simulink model "Simulation_ipmsm_velocity_control"  (R2023a)
settings: Solver=FixedStepDiscrete  StartTime=0.0  StopTime=2  FixedStep=Ts  RelTol=1e-3  EnableMultiTasking=on
PreLoadFcn:
  | ee_ipmsm_velocity_control_data;
StopFcn:
  | ee_addSimlogTimeStamp(bdroot)
undefined symbols (not defined in the file): Ld, Lq, p, psim, Ts, VDC_VECT, Vnom
libraries: nesl_utility x14, fl_lib x11, mcbcontrolslib x9, ee_lib x4, simulink x2, batteryecm_lib x1, eePmsmCurrentController x1, eeTransforms x1, eePmsmCurrentReferenceGen x1, eeVelocityController x1, eePwmGeneratorTwoLevel x1, SignalEditorBlockLib x1
(part 1 of 2)
CloseFcn:
  | try,close(h1_ee_ipmsm_velocity_control),end
  | clear h1_ee_ipmsm_velocity_control
  | 
  | clear simlog_ee_ipmsm_velocity_control
  | clear logsout_ee_ipmsm_velocity_control
  | 
  | clear Pmax Tmax p psim Ld Lq L0 Rs Jm
  | clear Cdc Vnom V1 AH0
  | clear Ts fsw Tsi Tso Kp_id Ki_id Kp_iq Ki_iq
  | clear numd_id dend_id numd_iq dend_iq
  | clear Kp_omega Ki_omega numd_omega dend_omega
  | clear ID_MAP IQ_MAP RPM_VECT TQ_VECT VDC_VECT
Description:
  | IPMSM Velocity Control
settings Model: Creator=The MathWorks, Inc.  LastModifiedBy=洲
settings SolverCC: AlgebraicLoopSolver=TrustRegion  MaxZcPerStep=1
settings DataIOCC: MaxDataPoints=210000  ReturnWorkspaceOutputs=off  SignalLoggingName=logsout_ee_ipmsm_velocity_control
settings OptimizationCC: ReuseModelBlockBuffer=off  LifeSpan=inf
settings DebuggingCC: MergeDetectMultiDrivingBlocksExec=none  UnconnectedInputMsg=warning  UnconnectedOutputMsg=warning  UnconnectedLineMsg=warning  SFUnexpectedBacktrackingDiag=warning  SFNoUnconditionalDefaultTransitionDiag=warning  SFExecutionAtInitializationDiag=none  ArithmeticOperatorsInVariantConditions=warning
settings ModelReferenceCC: EnableRefExpFcnMdlSchedulingChecks=on
settings SFSimCC: SimUseLocalCustomCode=off  CustomCodeUndefinedFunction=UseInterfaceOnly
settings RTWCC: RTWUseLocalCustomCode=off  DLArmComputeVersion=19.05
settings CodeAppCC: StateflowObjectComments=on
settings GRTTargetCC: TargetLangStandard=C89/C90 (ANSI)
settings ConfigComp: CovMetricSettings=dw  CovSaveCumulativeToWorkspaceVar=on  CovSaveSingleToWorkspaceVar=on  CovExternalEMLEnable=off
settings SimscapeCC: SimscapeNormalizeSystem=off  SimscapeLogType=all  SimscapeLogSimulationStatistics=on  SimscapeLogName=simlog_ee_ipmsm_velocity_control  SimscapeLogDataHistory=210000

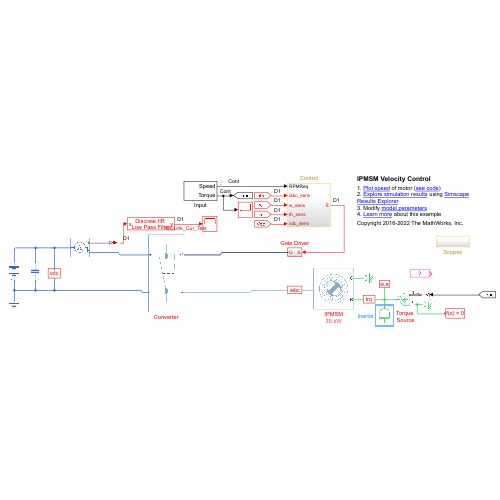
[thumbnail: Simulink's stored preview of the top-level diagram]
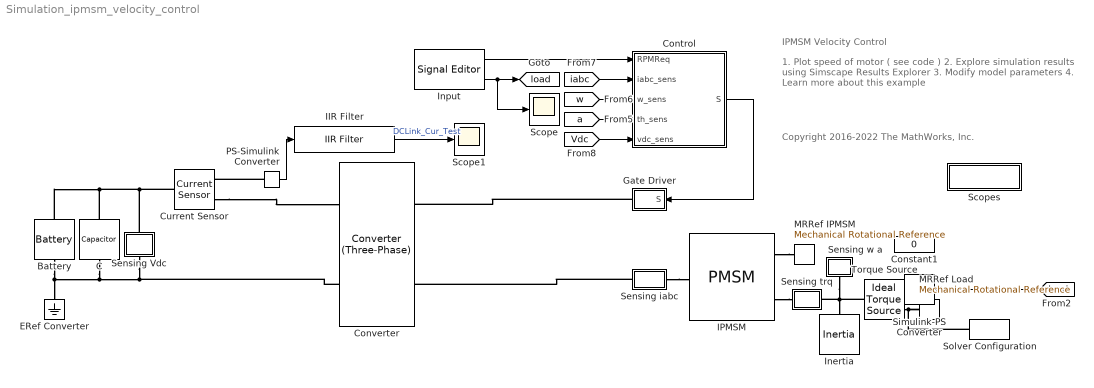
== system Simulation_ipmsm_velocity_control ==
  note: IPMSM Velocity Control
  note: 1. Plot speed of motor ( see code )
      | 2. Explore simulation results using Simscape Results Explorer
      | 3. Modify model parameters
      | 4. Learn more about this example
  note: Copyright 2016-2022 The MathWorks, Inc.
  Battery : batteryecm_lib/Battery  Vnom=Vnom V  prm_dir=1  R1_dis=2 Ohm  R1_ch=2 Ohm  R1=0.001 Ohm  prm_AH=1  AH=300 hr*A  V1=V1 V  AH1=100 hr*A  prm_R2=1  R2=2000 Ohm  Tmeas=298.15 K  charge_measurement_port=simscape.enum.battery.enable.no  prm_dyn=1  Rp1=0.005 Ohm  tau1=30 s  Rp2=0.005 Ohm  tau2=30 s  Rp3=0.005 Ohm  tau3=30 s  Rp4=0.005 Ohm  tau4=30 s  Rp5=0.005 Ohm  tau5=30 s  prm_fade=1  N_fade=100  AH_fade=45 hr*A  R1_fade=2.02 Ohm  R1_ch_fade=2.02 Ohm  V1_fade=10.35 V  prm_age=1  prm_age_OCV=1  OCV_age=0.9  SOC_age=60  Tmeas_age=298.15 K  delta_time_age_vec=[0] d  temperature_age_vec=[273] K  OCV_scaling_age=2.2134e6  OCV_offset_age=1.632e6  temp_exp_age=0.515833569 V  t_exp_age=0.75  Vnom_T2=12 V  R1_T2=2.2 Ohm  R1_T2_dis=2.2 Ohm  R1_T2_ch=2.2 Ohm  V1_T2=11.4 V  R2_T2=2200 Ohm  Rp1_T2=0.005 Ohm  tau1_T2=30 s  Rp2_T2=0.005 Ohm  tau2_T2=30 s  Rp3_T2=0.005 Ohm  tau3_T2=30 s  Rp4_T2=0.005 Ohm  tau4_T2=30 s  Rp5_T2=0.005 Ohm  tau5_T2=30 s  Tmeas2=273.15 K  thermal_port=simscape.enum.thermaleffects.omit  thermal_mass=30000 J/K  i_specify=off  i_priority=None  i=0 A  i_nominal_specify=off  i_nominal_unit=A  i_nominal_value=1  v_specify=off  v_priority=None  v=0 V  v_nominal_specify=off  v_nominal_unit=V  v_nominal_value=1  charge_specify=on  charge_priority=High  charge=AH0 hr*A  charge_nominal_specify=off  charge_nominal_unit=A*hr  charge_nominal_value=1  num_cycles_specify=off  num_cycles_priority=High  num_cycles=0  num_cycles_nominal_specify=off  num_cycles_nominal_unit=1  num_cycles_nominal_value=1  temperature_specify=off  temperature_priority=High  temperature=298.15 K  temperature_nominal_specify=off  temperature_nominal_unit=K  temperature_nominal_value=1
  C : fl_lib/Electrical/Electrical Elements/Capacitor  c=Cdc F  r=1e-6 Ohm  g=0 1/Ohm  i_specify=off  i_priority=None  i=0 A  i_nominal_specify=off  i_nominal_unit=A  i_nominal_value=1  v_specify=off  v_priority=None  v=0 V  v_nominal_specify=off  v_nominal_unit=V  v_nominal_value=1  vc_specify=on  vc_priority=None  vc=Vnom V  vc_nominal_specify=off  vc_nominal_unit=V  vc_nominal_value=1
  Constant1 : Constant  Value=0
  Control : Subsystem
  Converter : ee_lib/Semiconductors & Converters/Converters/Converter (Three-Phase)  port_option=ee.enum.threePhasePort.composite  device_type=3  K=0  Vf=0.8 V  Ron=0.001 Ohm  Rds=0.001 Ohm  Goff=1e-5 1/Ohm  Vgt=1 V  Vgt_off=-1 V  Ih=1 A  Vth=0.5 V  diode_param=2  diode_Vf=0.8 V  diode_Ron=0.001 Ohm  diode_Goff=1e-5 1/Ohm  diode_C=50 nF  diode_iRM=-235 A  diode_iF=300 A  diode_idot=-50 A/us  diode_trr_param=1  diode_trr_factor=3  diode_trr=15 us  diode_Qrr=1.5e+3 s*uA  snubber_type=0  Cs=1e-7 F  Rs=0.1 Ohm
  Current Sensor : fl_lib/Electrical/Electrical Sensors/Current Sensor
  ERef Converter : fl_lib/Electrical/Electrical Elements/Electrical Reference
  Gate Driver : Subsystem
  IIR Filter : mcbcontrolslib/IIR Filter  VariantControl=Low Pass Filter  VariantSelect=Low-pass  Filter_constant=0.001  advancedSettings=off  Ts=50e-6  cutOff_freq=3.1863
      settings: LibrarySourceBlock=mcbhdllib/Signal Management/IIR Filter
  IPMSM : ee_lib/Electromechanical/Permanent Magnet/PMSM  port_option=ee.enum.threePhasePort.composite  winding_type=ee.enum.statorconnection.wye  machine_param=ee.enum.pmsm.parameterization.constant  nPolePairs=p  pmflux_param=1  pm_flux_linkage=psim Wb  torque_constant=0.18 N*m/A  back_emf_constant=0.18 V/(rad/s)  stator_param=1  Ld=Ld H  Lq=Lq H  idVec=[-200, 0, 200] A  iqVec=[-200, 0, 200] A  LdMatrix=0.0002 * ones(3, 3) H  LqMatrix=0.0002 * ones(3, 3) H  PmMatrix=0.1 * ones(3, 3) Wb  ktMatrix=0.18 * ones(3, 3) N*m/A  keMatrix=0.18 * ones(3, 3) V/(rad/s)  L0=L0 H  Ls=0.0002 H  Lm=0.00002 H  Ms=0.00002 H  Rs=Rs Ohm  zero_sequence=ee.enum.park.zerosequence.exclude  axes_param=ee.enum.rotorangle.daxis  loss_param=ee.enum.ironloss.none  losses_oc=[0, 0, 0] W  losses_sc=[0, 0, 0] W  f_losses=60 Hz  Isc_losses=95 A  J=0 kg*m^2  lam=0 N*m/(rad/s)  i_d_specify=off  i_d_priority=None  i_d=0 A  i_d_nominal_specify=off  i_d_nominal_unit=A  i_d_nominal_value=1  i_q_specify=off  i_q_priority=None  i_q=0 A  i_q_nominal_specify=off  i_q_nominal_unit=A  i_q_nominal_value=1  torque_specify=off  torque_priority=None  torque=0 N*m  torque_nominal_specify=off  torque_nominal_unit=N*m  torque_nominal_value=1  angular_velocity_specify=on  angular_velocity_priority=None  angular_velocity=0 rpm  angular_velocity_nominal_specify=off  angular_velocity_nominal_unit=rpm  angular_velocity_nominal_value=1  angular_position_specify=on  angular_position_priority=High  angular_position=0 rad  angular_position_nominal_specify=off  angular_position_nominal_unit=deg  angular_position_nominal_value=1  alpha=3.93e-3 1/K  alpha_flux=-0.001 1/K  Tmeas=298.15 K  stator_thermal_mass=100 J/K  rotor_thermal_mass=200 J/K  Rm_percent_rotor=90  Rd_percent_rotor=30  temperatureA_specify=off  temperatureA_priority=High  temperatureA=25 degC  temperatureA_nominal_specify=off  temperatureA_nominal_unit=degC  temperatureA_nominal_value=1  temperatureB_specify=off  temperatureB_priority=High  temperatureB=25 degC  temperatureB_nominal_specify=off  temperatureB_nominal_unit=degC  temperatureB_nominal_value=1  temperatureC_specify=off  temperatureC_priority=High  temperatureC=25 degC  temperatureC_nominal_specify=off  temperatureC_nominal_unit=degC  temperatureC_nominal_value=1  temperatureR_specify=off  temperatureR_priority=High  temperatureR=25 degC  temperatureR_nominal_specify=off  temperatureR_nominal_unit=degC  temperatureR_nominal_value=1
      settings: AttributesFormatString=35 kW  InternalSimscapePortConfiguration="{\"Bottom\":[],\"Left\":[{\"id\":\"N\",\"label\":\"~\",\"type\":\"foundation.electrical.three_phase\"}],\"Right\":[{\"id\":\"R\",\"label\":\"R\",\"type\":\"foundation.mechanical.rotational.rotational\"},{\"id\":\"C\",\"label\":\"C\",\"type\":\"foundation.mechanical.rotational.rotational\"}],\"Top\":[]}"
  Inertia : fl_lib/Mechanical/Rotational Elements/Inertia  inertia=Jm kg*m^2  num_ports=foundation.enum.numPorts2.one  w_specify=on  w_priority=High  w=0 rpm  w_nominal_specify=off  w_nominal_unit=rad/s  w_nominal_value=1  t_specify=off  t_priority=High  t=0 N*m  t_nominal_specify=off  t_nominal_unit=N*m  t_nominal_value=1
  Input : SignalEditorBlockLib/Signal Editor  FileName=ee_ipmsm_velocity_control_Input.mat  ActiveScenario=Test_1  ActiveSignal=Torque  IsBus=off  OutputBusObjectStr=Bus: BusObject  SampleTime=0  OutputAfterFinalValue=Extrapolation  Unit=inherit  PreserveSignalName=on  ApplySigPropsToAllScenarios=on
  MRRef IPMSM : fl_lib/Mechanical/Rotational Elements/Mechanical Rotational Reference
  MRRef Load : fl_lib/Mechanical/Rotational Elements/Mechanical Rotational Reference
  PS-Simulink Converter : nesl_utility/PS-Simulink Converter  PhysicalDomain=network_engine_domain  SubClassName=ps_output  LeftPortType=input  RightPortType=output  PseudoPeriodic=off  Frequencies=[]  VectorFormat=inherit  Unit=inherit  AffineConversion=off
  Scope : Scope
  Scope1 : Scope
  Scopes : Subsystem
  Sensing Vdc : Subsystem
      mask Display: disp('vdc')
  Sensing trq : Subsystem
      mask Display: disp('trq')
  Sensing w a : Subsystem
      mask Display: disp('w,a')
  Sensing iabc : Subsystem
      mask Display: disp('iabc')
  Simulink-PS Converter : nesl_utility/Simulink-PS Converter  PhysicalDomain=network_engine_domain  SubClassName=ps_input  LeftPortType=input  RightPortType=output  PseudoPeriodic=off  Frequencies=[]  NoiseDistribution=none  NoiseParameters=[]  Unit=N*m  AffineConversion=off  FilteringAndDerivatives=zero  SimscapeFilterOrder=1  InputFilterTimeConstant=0.001  UdotUserProvided=1
  Solver Configuration : nesl_utility/Solver Configuration  PhysicalDomain=network_engine_domain  SubClassName=solver  LeftPortType=input  RightPortType=generic  Tones=[]  Harmonics=[]  SimulateNoise=off  Profile=off  UseLocalSampling=off  EnableSwitchedLinearOptims=on  FrequencyDomain=off  UseCCode=off  RelTol=0.001  AbsTol=1e-06  MinStep=1e-09  ToWorkspace=off  RevertToSquareIcSolve=off  NumHomotopyIterations=100  PhasorMode=off  PhasorModeNumHarmonics=1  ConsistencySolver=NEWTON_FTOL  IndexReductionMethod=DerivativeReplacement  DoDC=off  ResidualTolerance=1e-9  ConsistencyTolSource=GLOBAL  ConsistencyAbsTol=0.001  ConsistencyRelTol=0.001  ConsistencyTolFactor=0.001  UseLocalSolver=on  LocalSolverChoice=NE_BACKWARD_EULER_ADVANCER  ResolveIndetEquations=on  FunctionEvalNumThread=1  LocalSolverSampleTime=Ts  DoFixedCost=on  MaxNonlinIter=5  MaxModeIter=2  ComputeImpulses=off  ImpulseIterations=2  LinearAlgebra=auto  LinearAlgebraNumThread=0  EquationFormulation=NE_TIME_EF  DelaysMemoryBudget=1024  AutomaticFiltering=on  FilteringTimeConstant=0.001  PartitionStorageMethod=AS_NEEDED  PartitionMemoryBudget=1024  PartitionMethod=FAST
  Torque Source : fl_lib/Mechanical/Mechanical Sources/Ideal Torque Source
  tag scope: load=global
  wires:
  Control/1(S) -> Gate Driver/1(S)
  [Vdc] -> Control/5(vdc_sens)
  [iabc] -> Control/2(iabc_sens)
  [w] -> Control/3(w_sens)
  [a] -> Control/4(th_sens)
  Input/2 -> [load], Scope/1
  Input/1 -> Control/1(RPMReq)
  PS-Simulink Converter/1 -> IIR Filter/1
  IIR Filter/1 -> Scope1/1  "DCLink_Cur_Test"
  [load] -> Simulink-PS Converter/1
  connections:
  Sensing Vdc/LConn1 -- Current Sensor/LConn1 -- C/LConn1 -- Battery/LConn1
  Torque Source/LConn1 -- Sensing trq/RConn1 -- Inertia/LConn1 -- Sensing w a/LConn1
  Gate Driver/RConn1 -- Converter/LConn1
  Torque Source/RConn1 -- Simulink-PS Converter/RConn1
  Torque Source/RConn2 -- Solver Configuration/RConn1 -- MRRef Load/LConn1
  Sensing iabc/LConn1 -- Converter/LConn2
  Sensing iabc/RConn1 -- IPMSM/LConn1
  IPMSM/RConn2 -- MRRef IPMSM/LConn1
  IPMSM/RConn1 -- Sensing trq/LConn1
  Battery/RConn1 -- C/RConn1 -- Sensing Vdc/RConn1 -- Converter/RConn2 -- ERef Converter/LConn1
  Current Sensor/RConn2 -- Converter/RConn1
  PS-Simulink Converter/LConn1 -- Current Sensor/RConn1

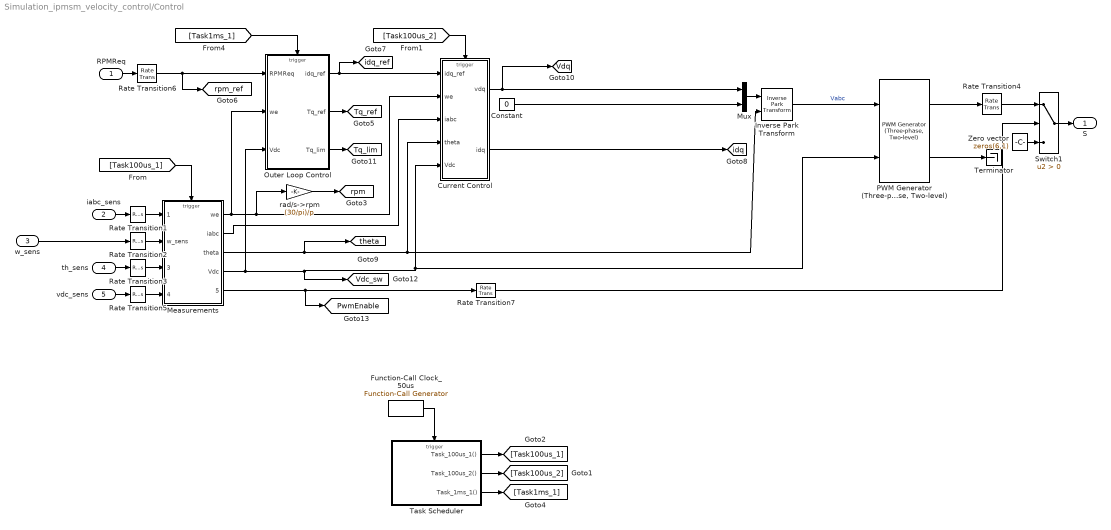
== system Simulation_ipmsm_velocity_control/Control ==
  RPMReq : Inport
  iabc_sens : Inport  Port=2
  w_sens : Inport  Port=3
  th_sens : Inport  Port=4
  vdc_sens : Inport  Port=5
  Constant : Constant  Value=0  SampleTime=-1
  Current Control : Subsystem
  Function-Call Clock_50us : simulink/Ports & Subsystems/Function-Call Generator  sample_time=5e-5  numberOfIterations=1  DisallowWideOutput=off
  Inverse Park Transform : eeTransforms/Inverse Park Transform  AxisAlignment=D-axis  PowerInvariant=off
  Measurements : Subsystem
  Mux : Mux  Inputs=2
  Outer Loop Control : Subsystem
  "PWM Generator (Three-phase, Two-level)" : eePwmGeneratorTwoLevel/PWM Generator (Three-phase, Two-level)  PWMMode=Continuous PWM (CPWM)  CPWMMode=SVM: space vector modulation  DPWMMode=60 DPWM: 60 degree discontinuous PWM  fsw=fsw  Ts=Ts
  Rate Transition{1..7} (7 alike) : RateTransition
  Switch1 : Switch  Criteria=u2 > Threshold  SaturateOnIntegerOverflow=off  InputSameDT=off
  Task Scheduler : Stateflow chart  TreatAsAtomicUnit=on
  Terminator : Terminator
  Zero vector : Constant  Value=zeros(6,1)
  rad/s->rpm : Gain  Gain=(30/pi)/p
  S : Outport  VectorParamsAs1DForOutWhenUnconnected=off
  tag scope: PwmEnable=global, Tq_lim=global, Tq_ref=global, Vdc_sw=global, Vdq=global, idq=global, idq_ref=global, rpm=global, rpm_ref=global, theta=global
  wires:
  [Task100us_1] -> Measurements/Trigger
  [Task100us_2] -> Current Control/Trigger
  Current Control/1(vdq) -> [Vdq], Mux/1
  Measurements/2(iabc) -> Current Control/3(iabc)
  Measurements/3(theta) -> [theta], Inverse Park Transform/2, Current Control/4(theta)
  "PWM Generator (Three-phase, Two-level)"/1 -> Rate Transition4/1
  Inverse Park Transform/1 -> "PWM Generator (Three-phase, Two-level)"/1  "Vabc"
  iabc_sens/1 -> Rate Transition1/1
  w_sens/1 -> Rate Transition2/1
  th_sens/1 -> Rate Transition3/1
  vdc_sens/1 -> Rate Transition5/1
  Outer Loop Control/1(idq_ref) -> [idq_ref], Current Control/1(idq_ref)
  RPMReq/1 -> Rate Transition6/1
  "PWM Generator (Three-phase, Two-level)"/2 -> Terminator/1
  Rate Transition1/1 -> Measurements/1(iabc_sens)
  Rate Transition2/1 -> Measurements/2(w_sens)
  Rate Transition3/1 -> Measurements/3(th_sens)
  Rate Transition5/1 -> Measurements/4(Vdc_sens)
  Rate Transition6/1 -> [rpm_ref], Outer Loop Control/1(RPMReq)
  Measurements/4(Vdc) -> [Vdc_sw], "PWM Generator (Three-phase, Two-level)"/2, Current Control/5(Vdc), Outer Loop Control/3(Vdc)
  Function-Call Clock_50us/1 -> Task Scheduler/Trigger
  Task Scheduler/3(Task_1ms_1()) -> [Task1ms_1]
  Task Scheduler/2(Task_100us_2()) -> [Task100us_2]
  Task Scheduler/1(Task_100us_1()) -> [Task100us_1]
  Outer Loop Control/2(Tq_ref) -> [Tq_ref]
  Measurements/1(we) -> Current Control/2(we), rad/s->rpm/1, Outer Loop Control/2(we)
  rad/s->rpm/1 -> [rpm]
  Current Control/2(idq) -> [idq]
  Outer Loop Control/3(Tq_lim) -> [Tq_lim]
  Switch1/1 -> S/1
  Rate Transition4/1 -> Switch1/1
  Measurements/5(PwmEnable) -> [PwmEnable], Rate Transition7/1
  Zero vector/1 -> Switch1/3
  Rate Transition7/1 -> Switch1/2
  [Task1ms_1] -> Outer Loop Control/Trigger
  Mux/1 -> Inverse Park Transform/1
  Constant/1 -> Mux/2

== system Simulation_ipmsm_velocity_control/Gate Driver ==
  S : Inport
  Demux : Demux  Outputs=6
  Simulink-PS Converter{1..6} (6 alike) : nesl_utility/Simulink-PS Converter  PhysicalDomain=network_engine_domain  SubClassName=ps_input  LeftPortType=input  RightPortType=output  PseudoPeriodic=off  Frequencies=[]  NoiseDistribution=none  NoiseParameters=[]  Unit=1  AffineConversion=off  FilteringAndDerivatives=zero  SimscapeFilterOrder=1  InputFilterTimeConstant=0.001  UdotUserProvided=1
  Six-Pulse Gate Multiplexer : ee_lib/Semiconductors & Converters/Converters/Six-Pulse Gate Multiplexer  port_option=ee.enum.controlport.ps
  G : PMIOPort  Side=Right
  wires:
  Demux/1 -> Simulink-PS Converter1/1
  S/1 -> Demux/1
  Demux/4 -> Simulink-PS Converter4/1
  Demux/2 -> Simulink-PS Converter2/1
  Demux/3 -> Simulink-PS Converter3/1
  Demux/5 -> Simulink-PS Converter5/1
  Demux/6 -> Simulink-PS Converter6/1
  connections:
  Six-Pulse Gate Multiplexer/RConn1 -- G/RConn1
  Simulink-PS Converter1/RConn1 -- Six-Pulse Gate Multiplexer/LConn1
  Simulink-PS Converter3/RConn1 -- Six-Pulse Gate Multiplexer/LConn3
  Simulink-PS Converter5/RConn1 -- Six-Pulse Gate Multiplexer/LConn5
  Simulink-PS Converter6/RConn1 -- Six-Pulse Gate Multiplexer/LConn6
  Simulink-PS Converter4/RConn1 -- Six-Pulse Gate Multiplexer/LConn4
  Simulink-PS Converter2/RConn1 -- Six-Pulse Gate Multiplexer/LConn2

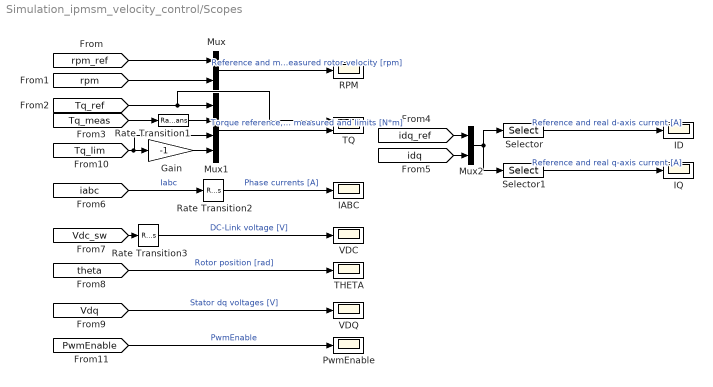
== system Simulation_ipmsm_velocity_control/Scopes ==
  Gain : Gain  Gain=-1
  IABC : Scope
  ID : Scope
  IQ : Scope
  Mux : Mux  Inputs=2
  Mux1 : Mux
  Mux2 : Mux  Inputs=2
  PwmEnable : Scope
  RPM : Scope
  Rate Transition1 : RateTransition
  Rate Transition2 : RateTransition  OutPortSampleTime=1e-4
  Rate Transition3 : RateTransition  OutPortSampleTime=1e-4
  Selector : Selector  InputPortWidth=4  IndexOptions=Index vector (dialog)  Indices=[1 3]  OutputSizes=1
  Selector1 : Selector  InputPortWidth=4  IndexOptions=Index vector (dialog)  Indices=[2 4]  OutputSizes=1
  THETA : Scope
  TQ : Scope  NumInputPorts=2
  VDC : Scope
  VDQ : Scope
  wires:
  [rpm] -> Mux/2
  Selector1/1 -> IQ/1  "Reference and real q-axis current [A]"
  Mux2/1 -> Selector1/1, Selector/1
  Gain/1 -> Mux1/4
  Rate Transition3/1 -> VDC/1  "DC-Link voltage [V]"
  [Vdc_sw] -> Rate Transition3/1
  [idq_ref] -> Mux2/1
  [PwmEnable] -> PwmEnable/1  "PwmEnable"
  [Tq_ref] -> TQ/1, Mux1/1
  Rate Transition2/1 -> IABC/1  "Phase currents [A]"
  [idq] -> Mux2/2
  [rpm_ref] -> Mux/1
  [iabc] -> Rate Transition2/1  "Iabc"
  [Tq_meas] -> Rate Transition1/1
  [Vdq] -> VDQ/1  "Stator dq voltages [V]"
  Selector/1 -> ID/1  "Reference and real d-axis current [A]"
  [Tq_lim] -> Mux1/3, Gain/1
  Mux1/1 -> TQ/2  "Torque reference, measured and limits [N*m]"
  [theta] -> THETA/1  "Rotor position [rad]"
  Rate Transition1/1 -> Mux1/2
  Mux/1 -> RPM/1  "Reference and measured rotor velocity [rpm]"

== system Simulation_ipmsm_velocity_control/Sensing Vdc ==
  PS-Simulink Converter4 : nesl_utility/PS-Simulink Converter  PhysicalDomain=network_engine_domain  SubClassName=ps_output  LeftPortType=input  RightPortType=output  PseudoPeriodic=off  Frequencies=[]  VectorFormat=1-D array  Unit=V  AffineConversion=off
  Voltage Sensor : fl_lib/Electrical/Electrical Sensors/Voltage Sensor
  + : PMIOPort  Side=Left
  - : PMIOPort  Port=2  Side=Right
  tag scope: Vdc=global
  wires:
  PS-Simulink Converter4/1 -> [Vdc]
  connections:
  Voltage Sensor/LConn1 -- +/RConn1
  Voltage Sensor/RConn2 -- -/RConn1
  PS-Simulink Converter4/LConn1 -- Voltage Sensor/RConn1

== system Simulation_ipmsm_velocity_control/Sensing trq ==
  PS-Simulink Converter3 : nesl_utility/PS-Simulink Converter  PhysicalDomain=network_engine_domain  SubClassName=ps_output  LeftPortType=input  RightPortType=output  PseudoPeriodic=off  Frequencies=[]  VectorFormat=1-D array  Unit=N*m  AffineConversion=off
  Torque Sensor : fl_lib/Mechanical/Mechanical Sensors/Ideal Torque Sensor
  R : PMIOPort  Side=Left
  C : PMIOPort  Port=2  Side=Right
  tag scope: Tq_meas=global
  wires:
  PS-Simulink Converter3/1 -> [Tq_meas]
  connections:
  Torque Sensor/RConn1 -- C/RConn1
  Torque Sensor/RConn2 -- PS-Simulink Converter3/LConn1
  Torque Sensor/LConn1 -- R/RConn1

== system Simulation_ipmsm_velocity_control/Sensing w a ==
  MRRef : fl_lib/Mechanical/Rotational Elements/Mechanical Rotational Reference
  Motion Sensor : fl_lib/Mechanical/Mechanical Sensors/Ideal Rotational Motion Sensor  reference=foundation.enum.MeasurementReference.difference  acceleration_port=false  velocity_port=true  position_port=true  wrap_angle=simscape.enum.onoff.off  offset=0 deg
  PS-Simulink Converter1 : nesl_utility/PS-Simulink Converter  PhysicalDomain=network_engine_domain  SubClassName=ps_output  LeftPortType=input  RightPortType=output  PseudoPeriodic=off  Frequencies=[]  VectorFormat=1-D array  Unit=rad/s  AffineConversion=off
  PS-Simulink Converter2 : nesl_utility/PS-Simulink Converter  PhysicalDomain=network_engine_domain  SubClassName=ps_output  LeftPortType=input  RightPortType=output  PseudoPeriodic=off  Frequencies=[]  VectorFormat=1-D array  Unit=rad  AffineConversion=off
  Scope : Scope
  R : PMIOPort  Side=Left
  tag scope: a=global, w=global
  wires:
  PS-Simulink Converter1/1 -> [w]  "eSpd"
  PS-Simulink Converter2/1 -> [a]
  connections:
  R/RConn1 -- Motion Sensor/LConn1
  Motion Sensor/RConn2 -- PS-Simulink Converter1/LConn1
  MRRef/LConn1 -- Motion Sensor/RConn1
  Motion Sensor/RConn3 -- PS-Simulink Converter2/LConn1

== system Simulation_ipmsm_velocity_control/Sensing iabc ==
  Current Sensor : ee_lib/Sensors & Transducers/Current Sensor (Three-Phase)
  PS-Simulink Converter : nesl_utility/PS-Simulink Converter  PhysicalDomain=network_engine_domain  SubClassName=ps_output  LeftPortType=input  RightPortType=output  PseudoPeriodic=off  Frequencies=[]  VectorFormat=1-D array  Unit=A  AffineConversion=off
  1 : PMIOPort  Side=Left
  2 : PMIOPort  Port=2  Side=Right
  tag scope: iabc=global
  wires:
  PS-Simulink Converter/1 -> [iabc]
  connections:
  1/RConn1 -- Current Sensor/LConn1
  2/RConn1 -- Current Sensor/RConn2
  Current Sensor/RConn1 -- PS-Simulink Converter/LConn1

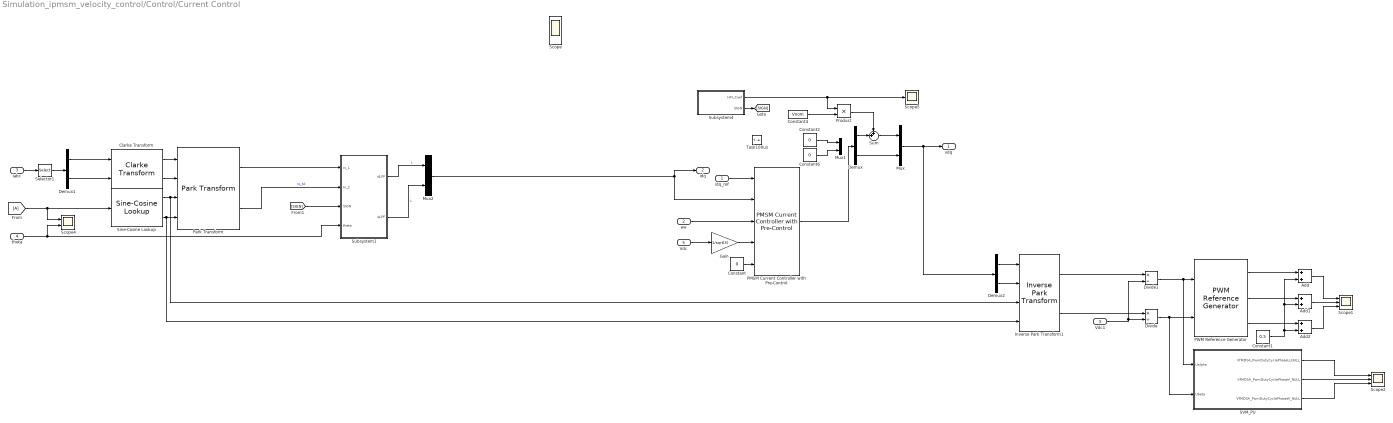
== system Simulation_ipmsm_velocity_control/Control/Current Control ==
  idq_ref : Inport
  we : Inport  Port=2
  iabc : Inport  Port=3
  theta : Inport  Port=4
  Vdc : Inport  Port=5
  Task100us : TriggerPort  TriggerType=function-call  VariantControl=Variant  PortDimensions=1
  Add : Sum
  Add1 : Sum
  Add2 : Sum
  Clarke Transform : mcbcontrolslib/Clarke Transform  VariantControl=Variant2
      settings: LibrarySourceBlock=mcblib/Controls/Math Transforms/Clarke Transform
  Constant : Constant  Value=0  SampleTime=-1
  Constant1 : Constant  Value=0.5
  Constant2 : Constant  Value=0
  Constant4 : Constant  Value=Vnom
  Constant6 : Constant  Value=0
  Demux : Demux  Outputs=2
  Demux1 : Demux  Outputs=2
  Demux2 : Demux  Outputs=2
  Divide : Product  Inputs=*/
  Divide1 : Product  Inputs=*/
  From : From
  Gain : Gain  Gain=1/sqrt(3)
  Inverse Park Transform1 : mcbcontrolslib/Inverse Park Transform  AxisAlignment=D-axis
      settings: LibrarySourceBlock=mcblib/Controls/Math Transforms/Inverse Park Transform
  Mux : Mux  Inputs=2
  Mux1 : Mux  Inputs=2
  Mux2 : Mux  Inputs=2
  PMSM Current Controller with Pre-Control : eePmsmCurrentController/PMSM Current Controller with Pre-Control  Kp_id=Kp_id  Ki_id=Ki_id  Kaw_id=1  Kp_iq=Kp_iq  Ki_iq=Ki_iq  Kaw_iq=1  Ts=-1  Tsd=Tsi  AxisPrio=D-axis  ActZC=on  ActFF=on  idVect=[-200, 0, 200]  iqVect=[-200, 0, 200]  LdMatrix=Ld * ones(3, 3)  LqMatrix=Lq * ones(3, 3)  psimMatrix=psim * ones(3, 3)
  PWM Reference Generator : mcbcontrolslib/PWM Reference Generator  inSignal=Valphabeta  modType=SVM: space vector modulation
      settings: LibrarySourceBlock=mcblib/Controls/Math Transforms/PWM Reference Generator
  Park Transform : mcbcontrolslib/Park Transform  AxisAlignment=D-axis
      settings: LibrarySourceBlock=mcblib/Controls/Math Transforms/Park Transform
  Product : Product
  SVM_PU : Subsystem  TreatAsAtomicUnit=on  RTWFcnName=SVPWM_Calc
      settings: RTWSystemCode=Nonreusable function  RTWFcnNameOpts=User specified
  Scope : Scope  NumInputPorts=4
  Scope1 : Scope  NumInputPorts=3
  Scope2 : Scope  NumInputPorts=3
  Scope4 : Scope  NumInputPorts=2
  Scope5 : Scope
  Selector1 : Selector  InputPortWidth=3  IndexOptions=Index vector (dialog)  Indices=[1 2]  OutputSizes=1
  Sine-Cosine Lookup : mcbcontrolslib/Sine-Cosine Lookup  AngleInput=Radians  N_points=4095
      settings: LibrarySourceBlock=mcblib/Controls/Math Transforms/Sine-Cosine Lookup
  Subsystem1 : Subsystem
  Subsystem4 : Subsystem
  Sum : Sum  Inputs=++|
  Vdc1 : InportShadow  Port=5
  vdq : Outport  VectorParamsAs1DForOutWhenUnconnected=off
  idq : Outport  Port=2  VectorParamsAs1DForOutWhenUnconnected=off
  wires:
  Vdc/1 -> Gain/1
  we/1 -> PMSM Current Controller with Pre-Control/3
  idq_ref/1 -> PMSM Current Controller with Pre-Control/1
  Constant/1 -> PMSM Current Controller with Pre-Control/5
  Mux2/1 -> idq/1, PMSM Current Controller with Pre-Control/2
  Gain/1 -> PMSM Current Controller with Pre-Control/4
  iabc/1 -> Selector1/1
  Selector1/1 -> Demux1/1
  Demux1/1 -> Clarke Transform/1
  Demux1/2 -> Clarke Transform/2
  Clarke Transform/1 -> Park Transform/1
  Clarke Transform/2 -> Park Transform/2
  Sine-Cosine Lookup/1 -> Inverse Park Transform1/3, Park Transform/3
  Sine-Cosine Lookup/2 -> Inverse Park Transform1/4, Park Transform/4
  Mux/1 -> vdq/1, Demux2/1
  Park Transform/1 -> Subsystem1/1(In_1)
  Park Transform/2 -> Subsystem1/2(In_2)  "Iq_bk"
  From/1 -> Scope4/1, Sine-Cosine Lookup/1
  Demux2/1 -> Inverse Park Transform1/1
  Demux2/2 -> Inverse Park Transform1/2
  Vdc1/1 -> Divide1/2, Divide/2
  Inverse Park Transform1/1 -> Divide1/1
  Divide1/1 -> SVM_PU/1(Ualpha), PWM Reference Generator/1
  Divide/1 -> PWM Reference Generator/2, SVM_PU/2(Ubeta)
  Inverse Park Transform1/2 -> Divide/1
  PWM Reference Generator/1 -> Add/1
  PWM Reference Generator/2 -> Add1/1
  PWM Reference Generator/3 -> Add2/1
  Constant1/1 -> Add/2, Add1/2, Add2/2
  Add/1 -> Scope1/1
  Add1/1 -> Scope1/2
  Add2/1 -> Scope1/3
  SVM_PU/2(VfMDSA_PwmDutyCyclePhaseV_NULL) -> Scope2/2
  SVM_PU/1(VfMDSA_PwmDutyCyclePhaseU_NULL) -> Scope2/1
  SVM_PU/3(VfMDSA_PwmDutyCyclePhaseW_NULL) -> Scope2/3
  Product/1 -> Sum/1
  Constant4/1 -> Product/2
  Subsystem4/1(HFI_Coef) -> Scope5/1, Product/1
  theta/1 -> Subsystem1/4(theta), Scope4/2
  Sum/1 -> Mux/1
  Demux/1 -> Sum/2
  Demux/2 -> Mux/2
  Constant2/1 -> Mux1/1
  Constant6/1 -> Mux1/2
  PMSM Current Controller with Pre-Control/1 -> Demux/1
  Subsystem1/1(dLPF) -> Mux2/1  "L"
  Subsystem1/2(qLPF) -> Mux2/2  "L"
  Subsystem4/2(SIGN) -> [SIGN]
  [SIGN] -> Subsystem1/3(SIGN)

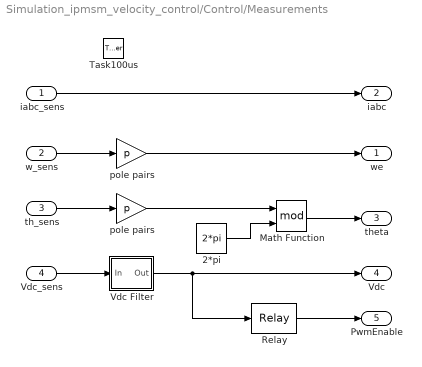
== system Simulation_ipmsm_velocity_control/Control/Measurements ==
  iabc_sens : Inport
  w_sens : Inport  Port=2
  th_sens : Inport  Port=3
  Vdc_sens : Inport  Port=4
  Task100us : TriggerPort  TriggerType=function-call  VariantControl=Variant  PortDimensions=1
  2*pi : Constant  Value=2*pi  SampleTime=-1
  Math Function : Math  Operator=mod  SignedPower=on
  Relay : Relay  OnSwitchValue=VDC_VECT(1)  OffSwitchValue=0.5*VDC_VECT(1)
  Vdc Filter : Subsystem  mask(Discrete first-order filter (Low-pass)){T=0.005, Ts=1e-4}
      mask prompts: T "Time constant (s):"; Ts "Sample time (s):"
      mask help: This block implements a discrete low-pass filter. To calculate the coefficients, the block discretises a continuous low-pass filter using the Tustin method.
      mask init:
      | num = [ Ts/(2*T + Ts), Ts/(2*T + Ts)];
      | den = [ 1, -(2*T - Ts)/(2*T + Ts)];
  pole pairs : Gain  Gain=p
  "pole pairs " : Gain  Gain=p
  we : Outport  VectorParamsAs1DForOutWhenUnconnected=off
  iabc : Outport  Port=2  VectorParamsAs1DForOutWhenUnconnected=off
  theta : Outport  Port=3  VectorParamsAs1DForOutWhenUnconnected=off
  Vdc : Outport  Port=4  VectorParamsAs1DForOutWhenUnconnected=off
  PwmEnable : Outport  Port=5  VectorParamsAs1DForOutWhenUnconnected=off
  wires:
  pole pairs/1 -> we/1
  Vdc_sens/1 -> Vdc Filter/1(In)
  th_sens/1 -> "pole pairs "/1
  w_sens/1 -> pole pairs/1
  iabc_sens/1 -> iabc/1
  "pole pairs "/1 -> Math Function/1
  2*pi/1 -> Math Function/2
  Math Function/1 -> theta/1
  Relay/1 -> PwmEnable/1
  Vdc Filter/1(Out) -> Relay/1, Vdc/1

== system Simulation_ipmsm_velocity_control/Control/Outer Loop Control ==
  RPMReq : Inport
  we : Inport  Port=2
  Vdc : Inport  Port=3
  Task1ms : TriggerPort  TriggerType=function-call  VariantControl=Variant  PortDimensions=1
  Constant : Constant  Value=0  SampleTime=-1
  PMSM Current Reference Generator : eePmsmCurrentReferenceGen/PMSM Current Reference Generator  Vnom=Vnom  Pmax=Pmax  Tmax=Tmax  Ts=-1  RefType=Lookup-table based  rpmVec=RPM_VECT  TqVec=TQ_VECT  VdcVec=VDC_VECT  PWMMode=SVM: space vector modulation  ModFactor=1  idMatrix=ID_MAP  iqMatrix=IQ_MAP  p=8  psim=0.04  Ld=0.00024  Lq=0.00029  Rs=0.01  RefExpEnable=0
  Velocity Controller : eeVelocityController/Velocity Controller  CtrlType=P-PI control  Kp_w=Kp_omega  Ki_w=Ki_omega  Kv_w=Kp_omega  Kaw_w=100  Ts=-1  Tsd=Tso  ActZC=on
  elec->mech : Gain  Gain=1/p
  rpm->rad/s : Gain  Gain=(pi/30)
  idq_ref : Outport  VectorParamsAs1DForOutWhenUnconnected=off
  Tq_ref : Outport  Port=2  VectorParamsAs1DForOutWhenUnconnected=off
  Tq_lim : Outport  Port=3  VectorParamsAs1DForOutWhenUnconnected=off
  wires:
  rpm->rad/s/1 -> Velocity Controller/1
  Velocity Controller/1 -> PMSM Current Reference Generator/1
  RPMReq/1 -> rpm->rad/s/1
  we/1 -> elec->mech/1
  Vdc/1 -> PMSM Current Reference Generator/3
  PMSM Current Reference Generator/1 -> idq_ref/1
  PMSM Current Reference Generator/2 -> Tq_ref/1, Velocity Controller/3
  PMSM Current Reference Generator/3 -> Tq_lim/1
  elec->mech/1 -> PMSM Current Reference Generator/2, Velocity Controller/2
  Constant/1 -> Velocity Controller/4

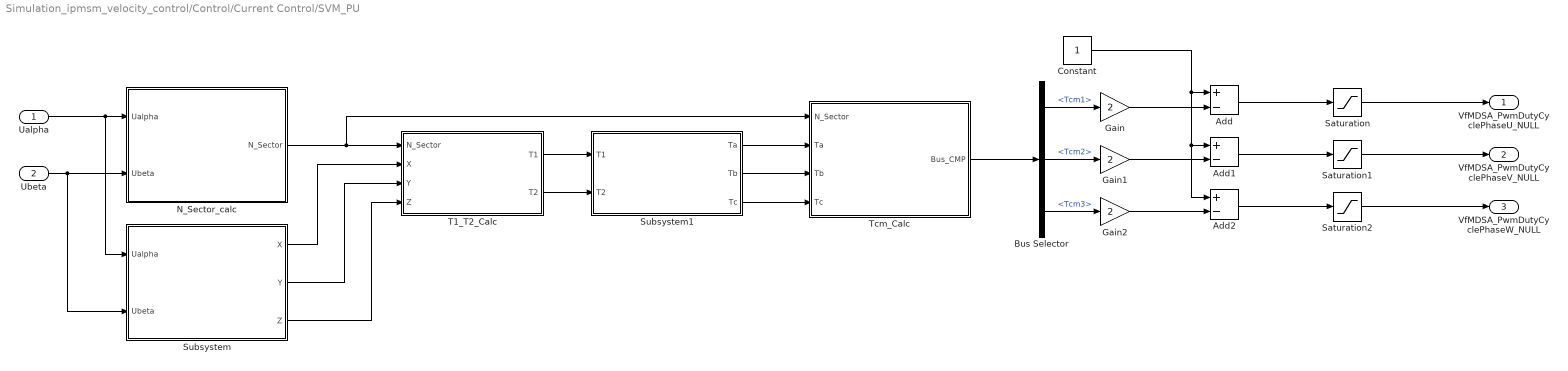
== system Simulation_ipmsm_velocity_control/Control/Current Control/SVM_PU ==
  Ualpha : Inport
  Ubeta : Inport  Port=2
  Add : Sum  Inputs=+-
  Add1 : Sum  Inputs=+-
  Add2 : Sum  Inputs=+-
  Bus Selector : BusSelector  OutputSignals=Tcm1,Tcm2,Tcm3
  Constant : Constant  OutDataTypeStr=single
  Gain : Gain  Gain=2
  Gain1 : Gain  Gain=2
  Gain2 : Gain  Gain=2
  N_Sector_calc : Subsystem
  Saturation : Saturate  UpperLimit=1  LowerLimit=0
  Saturation1 : Saturate  UpperLimit=1  LowerLimit=0
  Saturation2 : Saturate  UpperLimit=1  LowerLimit=0
  Subsystem : Subsystem
  Subsystem1 : Subsystem
  T1_T2_Calc : Subsystem
  Tcm_Calc : Subsystem
  VfMDSA_PwmDutyCyclePhaseU_NULL : Outport  OutMin=0  OutMax=1
  VfMDSA_PwmDutyCyclePhaseV_NULL : Outport  Port=2  OutMin=0  OutMax=1
  VfMDSA_PwmDutyCyclePhaseW_NULL : Outport  Port=3  OutMin=0  OutMax=1
  wires:
  Ualpha/1 -> Subsystem/1(Ualpha), N_Sector_calc/1(Ualpha)
  Ubeta/1 -> Subsystem/2(Ubeta), N_Sector_calc/2(Ubeta)
  N_Sector_calc/1(N_Sector) -> Tcm_Calc/1(N_Sector), T1_T2_Calc/1(N_Sector)
  Subsystem/1(X) -> T1_T2_Calc/2(X)
  Subsystem/2(Y) -> T1_T2_Calc/3(Y)
  Subsystem/3(Z) -> T1_T2_Calc/4(Z)
  Subsystem1/1(Ta) -> Tcm_Calc/2(Ta)
  Subsystem1/2(Tb) -> Tcm_Calc/3(Tb)
  Subsystem1/3(Tc) -> Tcm_Calc/4(Tc)
  Tcm_Calc/1(Bus_CMP) -> Bus Selector/1
  T1_T2_Calc/1(T1) -> Subsystem1/1(T1)
  T1_T2_Calc/2(T2) -> Subsystem1/2(T2)
  Bus Selector/1 -> Gain/1  "<Tcm1>"
  Bus Selector/2 -> Gain1/1  "<Tcm2>"
  Bus Selector/3 -> Gain2/1  "<Tcm3>"
  Constant/1 -> Add2/1, Add1/1, Add/1
  Gain/1 -> Add/2
  Gain1/1 -> Add1/2
  Gain2/1 -> Add2/2
  Add/1 -> Saturation/1
  Add1/1 -> Saturation1/1
  Add2/1 -> Saturation2/1
  Saturation/1 -> VfMDSA_PwmDutyCyclePhaseU_NULL/1
  Saturation1/1 -> VfMDSA_PwmDutyCyclePhaseV_NULL/1
  Saturation2/1 -> VfMDSA_PwmDutyCyclePhaseW_NULL/1

== system Simulation_ipmsm_velocity_control/Control/Current Control/Subsystem1 ==
  In_1 : Inport
  In_2 : Inport  Port=2
  SIGN : Inport  Port=3
  theta : Inport  Port=4
  Inverse Park Transform : mcbcontrolslib/Inverse Park Transform  AxisAlignment=D-axis
      settings: LibrarySourceBlock=mcblib/Controls/Math Transforms/Inverse Park Transform
  Scope : Scope  NumInputPorts=3
  Sine-Cosine Lookup : mcbcontrolslib/Sine-Cosine Lookup  AngleInput=Radians  N_points=4095
      settings: LibrarySourceBlock=mcblib/Controls/Math Transforms/Sine-Cosine Lookup
  Subsystem : Subsystem
  Subsystem2 : Subsystem
  Subsystem3 : Subsystem
  atan2 : mcbcontrolslib/atan2  outputUnit=Radians
      settings: LibrarySourceBlock=mcblib/Controls/Math Transforms/atan2
  dLPF : Outport
  qLPF : Outport  Port=2
  wires:
  Subsystem2/1(LPF) -> dLPF/1
  Subsystem3/2(LPF) -> qLPF/1
  In_1/1 -> Subsystem2/1(In_1)
  In_2/1 -> Subsystem3/1(In_2)
  Subsystem2/2(HPF) -> Subsystem/1(dHPF)
  Subsystem3/1(HPF) -> Subsystem/2(qHPF)
  SIGN/1 -> Subsystem/3(SIGN)
  Subsystem/1(delta_Id) -> Inverse Park Transform/1
  Subsystem/2(delta_Iq) -> Inverse Park Transform/2
  Sine-Cosine Lookup/2 -> Inverse Park Transform/4
  Sine-Cosine Lookup/1 -> Inverse Park Transform/3
  theta/1 -> Sine-Cosine Lookup/1
  Inverse Park Transform/1 -> Scope/1, atan2/1
  Inverse Park Transform/2 -> atan2/2, Scope/2
  atan2/1 -> Scope/3

== system Simulation_ipmsm_velocity_control/Control/Current Control/Subsystem4 ==
  Subsystem : Subsystem
  HFI_Coef : Outport
  SIGN : Outport  Port=2
  wires:
  Subsystem/1(HFI_Coef) -> HFI_Coef/1
  Subsystem/2(SIGN) -> SIGN/1

== system Simulation_ipmsm_velocity_control/Control/Measurements/Vdc Filter ==
  In : Inport
  Discrete Transfer Fcn : DiscreteTransferFcn  Numerator=num  Denominator=den
  Out : Outport  VectorParamsAs1DForOutWhenUnconnected=off
  wires:
  Discrete Transfer Fcn/1 -> Out/1
  In/1 -> Discrete Transfer Fcn/1

== system Simulation_ipmsm_velocity_control/Control/Current Control/SVM_PU/N_Sector_calc ==
  Ualpha : Inport
  Ubeta : Inport  Port=2
  N_calc : Subsystem
  Uref_Calc : Subsystem
  N_Sector : Outport
  wires:
  Uref_Calc/2(Uref2) -> N_calc/2(Uref2)
  Ualpha/1 -> Uref_Calc/1(Ualpha)
  Ubeta/1 -> Uref_Calc/2(Ubeta)
  Uref_Calc/3(Uref3) -> N_calc/3(Uref3)
  N_calc/1(N_Sector) -> N_Sector/1
  Uref_Calc/1(Uref1) -> N_calc/1(Uref1)

== system Simulation_ipmsm_velocity_control/Control/Current Control/SVM_PU/Subsystem ==
  Ualpha : Inport
  Ubeta : Inport  Port=2
  Add1 : Sum
  Add2 : Sum  Inputs=-+
  ConstanT1 : Constant  Value=2  OutDataTypeStr=single
  ConstanT2 : Constant  Value=sqrt(3)/2  OutDataTypeStr=single
  Constant : Constant  Value=3/2  OutDataTypeStr=single
  ProducT1 : Product
  ProducT2 : Product
  Product : Product
  X : Outport
  Y : Outport  Port=2
  Z : Outport  Port=3
  wires:
  Ualpha/1 -> Product/1
  Constant/1 -> Product/2
  ProducT1/1 -> X/1
  ConstanT1/1 -> ProducT1/2
  Ubeta/1 -> ProducT2/1
  Add1/1 -> Y/1
  Product/1 -> Add2/1, Add1/1
  ProducT2/1 -> ProducT1/1, Add2/2, Add1/2
  ConstanT2/1 -> ProducT2/2
  Add2/1 -> Z/1

== system Simulation_ipmsm_velocity_control/Control/Current Control/SVM_PU/Subsystem1 ==
  T1 : Inport
  T2 : Inport  Port=2
  Add : Sum  Inputs=+--
  Add1 : Sum  Inputs=++-
  Add2 : Sum  Inputs=+++
  Constant : Constant  Value=1/4  OutDataTypeStr=single
  Gain1 : Gain  Gain=1/4
  Gain2 : Gain  Gain=1/4
  Ta : Outport
  Tb : Outport  Port=2
  Tc : Outport  Port=3
  wires:
  T1/1 -> Gain1/1
  T2/1 -> Gain2/1
  Constant/1 -> Add2/1, Add1/1, Add/1
  Add/1 -> Ta/1
  Gain1/1 -> Add2/2, Add1/2, Add/2
  Gain2/1 -> Add1/3, Add2/3, Add/3
  Add1/1 -> Tb/1
  Add2/1 -> Tc/1

== system Simulation_ipmsm_velocity_control/Control/Current Control/SVM_PU/T1_T2_Calc ==
  N_Sector : Inport
  X : Inport  Port=2
  Y : Inport  Port=3
  Z : Inport  Port=4
  Subsystem1 : Subsystem
  Subsystem2 : Subsystem
  T4_T6 : Subsystem  Commented=on
  T1 : Outport
  T2 : Outport  Port=2
  wires:
  X/1 -> Subsystem1/2(X)
  Z/1 -> Subsystem1/4(Z)
  N_Sector/1 -> Subsystem1/1(N_Sector)
  Y/1 -> Subsystem1/3(Y)
  Subsystem1/1(Bus_T4T6) -> Subsystem2/1(Bus_T4T6)
  Subsystem2/1(T1) -> T1/1
  Subsystem2/2(T2) -> T2/1

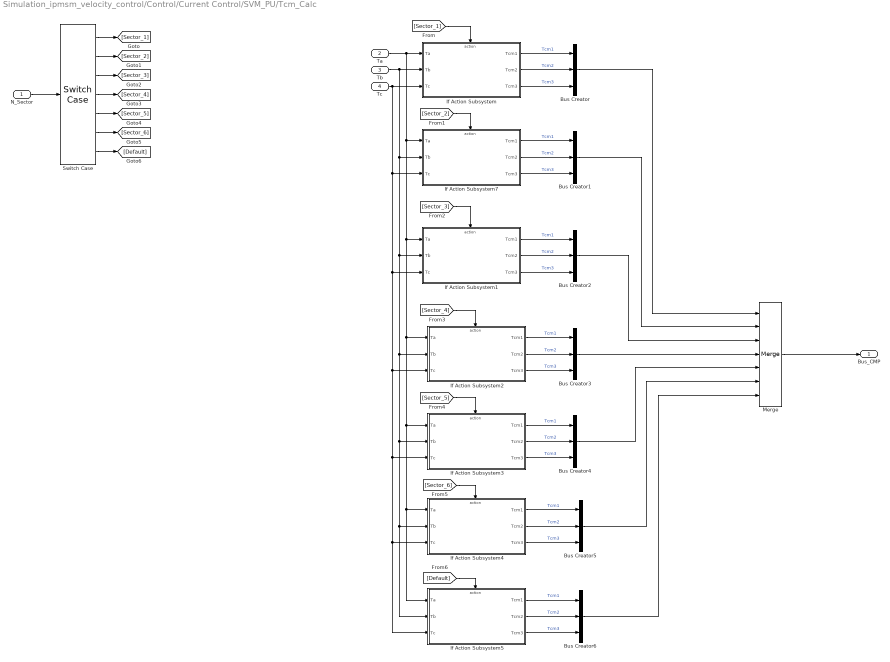
== system Simulation_ipmsm_velocity_control/Control/Current Control/SVM_PU/Tcm_Calc ==
  N_Sector : Inport
  Ta : Inport  Port=2
  Tb : Inport  Port=3
  Tc : Inport  Port=4
  Bus Creator{,1..6} (7 alike) : BusCreator  Inputs=3
  If Action Subsystem : Subsystem  TreatAsAtomicUnit=on
  If Action Subsystem1 : Subsystem  TreatAsAtomicUnit=on
  If Action Subsystem2 : Subsystem  TreatAsAtomicUnit=on
  If Action Subsystem3 : Subsystem  TreatAsAtomicUnit=on
  If Action Subsystem4 : Subsystem  TreatAsAtomicUnit=on
  If Action Subsystem5 : Subsystem  TreatAsAtomicUnit=on
  If Action Subsystem7 : Subsystem  TreatAsAtomicUnit=on
  Merge : Merge  Inputs=7
  Switch Case : SwitchCase  CaseConditions={1,2,3,4,5,6}
  Bus_CMP : Outport
  wires:
  Switch Case/1 -> [Sector_1]
  Switch Case/2 -> [Sector_2]
  Switch Case/4 -> [Sector_4]
  Switch Case/6 -> [Sector_6]
  Switch Case/3 -> [Sector_3]
  N_Sector/1 -> Switch Case/1
  Switch Case/7 -> [Default]
  Switch Case/5 -> [Sector_5]
  [Sector_1] -> If Action Subsystem/Action
  [Sector_2] -> If Action Subsystem7/Action
  [Sector_4] -> If Action Subsystem2/Action
  [Sector_3] -> If Action Subsystem1/Action
  [Sector_6] -> If Action Subsystem4/Action
  [Sector_5] -> If Action Subsystem3/Action
  [Default] -> If Action Subsystem5/Action
  Tb/1 -> If Action Subsystem5/2(Tb), If Action Subsystem4/2(Tb), If Action Subsystem3/2(Tb), If Action Subsystem2/2(Tb), If Action Subsystem1/2(Tb), If Action Subsystem7/2(Tb), If Action Subsystem/2(Tb)
  Tc/1 -> If Action Subsystem/3(Tc), If Action Subsystem5/3(Tc), If Action Subsystem4/3(Tc), If Action Subsystem3/3(Tc), If Action Subsystem2/3(Tc), If Action Subsystem1/3(Tc), If Action Subsystem7/3(Tc)
  Ta/1 -> If Action Subsystem5/1(Ta), If Action Subsystem4/1(Ta), If Action Subsystem3/1(Ta), If Action Subsystem2/1(Ta), If Action Subsystem1/1(Ta), If Action Subsystem7/1(Ta), If Action Subsystem/1(Ta)
  Merge/1 -> Bus_CMP/1
  If Action Subsystem/1(Tcm1) -> Bus Creator/1  "Tcm1"
  If Action Subsystem/2(Tcm2) -> Bus Creator/2  "Tcm2"
  If Action Subsystem/3(Tcm3) -> Bus Creator/3  "Tcm3"
  If Action Subsystem7/1(Tcm1) -> Bus Creator1/1  "Tcm1"
  If Action Subsystem7/3(Tcm3) -> Bus Creator1/3  "Tcm3"
  If Action Subsystem7/2(Tcm2) -> Bus Creator1/2  "Tcm2"
  If Action Subsystem1/1(Tcm1) -> Bus Creator2/1  "Tcm1"
  If Action Subsystem1/3(Tcm3) -> Bus Creator2/3  "Tcm3"
  If Action Subsystem1/2(Tcm2) -> Bus Creator2/2  "Tcm2"
  If Action Subsystem2/1(Tcm1) -> Bus Creator3/1  "Tcm1"
  If Action Subsystem2/3(Tcm3) -> Bus Creator3/3  "Tcm3"
  If Action Subsystem2/2(Tcm2) -> Bus Creator3/2  "Tcm2"
  If Action Subsystem3/1(Tcm1) -> Bus Creator4/1  "Tcm1"
  If Action Subsystem3/3(Tcm3) -> Bus Creator4/3  "Tcm3"
  If Action Subsystem3/2(Tcm2) -> Bus Creator4/2  "Tcm2"
  If Action Subsystem4/1(Tcm1) -> Bus Creator5/1  "Tcm1"
  If Action Subsystem4/3(Tcm3) -> Bus Creator5/3  "Tcm3"
  If Action Subsystem4/2(Tcm2) -> Bus Creator5/2  "Tcm2"
  If Action Subsystem5/1(Tcm1) -> Bus Creator6/1  "Tcm1"
  If Action Subsystem5/3(Tcm3) -> Bus Creator6/3  "Tcm3"
  If Action Subsystem5/2(Tcm2) -> Bus Creator6/2  "Tcm2"
  Bus Creator/1 -> Merge/1
  Bus Creator1/1 -> Merge/2
  Bus Creator2/1 -> Merge/3
  Bus Creator3/1 -> Merge/4
  Bus Creator4/1 -> Merge/5
  Bus Creator5/1 -> Merge/6
  Bus Creator6/1 -> Merge/7

== system Simulation_ipmsm_velocity_control/Control/Current Control/Subsystem1/Subsystem ==
  dHPF : Inport
  qHPF : Inport  Port=2
  SIGN : Inport  Port=3
  Add : Sum  Inputs=+-
  Add1 : Sum  Inputs=+-
  Delay : Delay  DelayLength=1
  Delay1 : Delay  DelayLength=1
  Product : Product
  Product1 : Product
  delta_Id : Outport
  delta_Iq : Outport  Port=2
  wires:
  dHPF/1 -> Delay/1, Add/1
  Delay/1 -> Add/2
  Add/1 -> Product/1
  qHPF/1 -> Delay1/1, Add1/1
  Delay1/1 -> Add1/2
  Add1/1 -> Product1/2
  SIGN/1 -> Product1/1, Product/2
  Product/1 -> delta_Id/1
  Product1/1 -> delta_Iq/1

== system Simulation_ipmsm_velocity_control/Control/Current Control/Subsystem1/Subsystem2 ==
  In_1 : Inport
  Add3 : Sum  Inputs=+-
  Constant7 : Constant  Value=0.0001
  Constant8 : Constant  Value=20
  HPF_Calc : Subsystem
  LPF : Outport
  HPF : Outport  Port=2
  wires:
  In_1/1 -> Add3/1, HPF_Calc/1(In1)
  Constant8/1 -> HPF_Calc/2(VfHpf_FilterCornerFreq_Hz)
  HPF_Calc/1(HPF) -> Add3/2, HPF/1
  Constant7/1 -> HPF_Calc/3(VfHpf_FilterTs_s)
  Add3/1 -> LPF/1

== system Simulation_ipmsm_velocity_control/Control/Current Control/Subsystem1/Subsystem3 ==
  In_2 : Inport
  Add3 : Sum  Inputs=+-
  Constant7 : Constant  Value=0.0001
  Constant8 : Constant  Value=20
  HPF_Calc : Subsystem
  HPF : Outport
  LPF : Outport  Port=2
  wires:
  In_2/1 -> Add3/1, HPF_Calc/1(In1)
  Constant8/1 -> HPF_Calc/2(VfHpf_FilterCornerFreq_Hz)
  HPF_Calc/1(HPF) -> Add3/2, HPF/1
  Constant7/1 -> HPF_Calc/3(VfHpf_FilterTs_s)
  Add3/1 -> LPF/1

== system Simulation_ipmsm_velocity_control/Control/Current Control/Subsystem4/Subsystem ==
  Compare To Constant : simulink/Logic and Bit Operations/Compare To Constant  relop=>  const=0  OutDataTypeStr=boolean
  Constant : Constant  OutDataTypeStr=single
  Constant1 : Constant  Value=-1  OutDataTypeStr=single
  Constant2 : Constant  Value=0.02
  Delay1 : Delay  DelayLength=1  InitialCondition=1
  Gain : Gain  Gain=-1
  Product1 : Product
  Switch : Switch  Criteria=u2 > Threshold  SaturateOnIntegerOverflow=off  InputSameDT=off
  HFI_Coef : Outport
  SIGN : Outport  Port=2
  wires:
  Constant/1 -> Switch/1
  Constant1/1 -> Switch/3
  Delay1/1 -> Gain/1, Compare To Constant/1  "HFI_Last_Coef"
  Gain/1 -> Product1/1, Delay1/1
  Compare To Constant/1 -> Switch/2
  Constant2/1 -> Product1/2
  Product1/1 -> HFI_Coef/1
  Switch/1 -> SIGN/1

== system Simulation_ipmsm_velocity_control/Control/Current Control/SVM_PU/N_Sector_calc/N_calc ==
  Uref1 : Inport
  Uref2 : Inport  Port=2
  Uref3 : Inport  Port=3
  Add : Sum  Inputs=+++
  ConstanT1 : Constant  Value=0  OutDataTypeStr=single
  Constant : Constant  OutDataTypeStr=single
  Gain : Gain
  Gain1 : Gain  Gain=2
  Gain2 : Gain  Gain=4
  Switch : Switch  Criteria=u2 > Threshold  SaturateOnIntegerOverflow=off  InputSameDT=off
  Switch1 : Switch  Criteria=u2 > Threshold  SaturateOnIntegerOverflow=off  InputSameDT=off
  Switch2 : Switch  Criteria=u2 > Threshold  SaturateOnIntegerOverflow=off  InputSameDT=off
  N_Sector : Outport
  wires:
  Uref1/1 -> Switch/2
  Uref2/1 -> Switch1/2
  Uref3/1 -> Switch2/2
  ConstanT1/1 -> Switch2/3, Switch/3, Switch1/3
  Constant/1 -> Switch2/1, Switch1/1, Switch/1
  Switch1/1 -> Gain1/1
  Switch/1 -> Gain/1
  Switch2/1 -> Gain2/1
  Add/1 -> N_Sector/1
  Gain/1 -> Add/1
  Gain1/1 -> Add/2
  Gain2/1 -> Add/3

== system Simulation_ipmsm_velocity_control/Control/Current Control/SVM_PU/N_Sector_calc/Uref_Calc ==
  Ualpha : Inport
  Ubeta : Inport  Port=2
  Add : Sum  Inputs=+-
  Add1 : Sum  Inputs=--
  ConstanT1 : Constant  Value=sqrt(1)/2  OutDataTypeStr=single
  Constant : Constant  Value=sqrt(3)/2  OutDataTypeStr=single
  ProducT1 : Product
  Product : Product
  Signal Copy : SignalConversion  OverrideOpt=off
  Uref1 : Outport
  Uref2 : Outport  Port=2
  Uref3 : Outport  Port=3
  wires:
  Ubeta/1 -> ProducT1/1, Signal Copy/1
  Signal Copy/1 -> Uref1/1
  Ualpha/1 -> Product/1
  Constant/1 -> Product/2
  ConstanT1/1 -> ProducT1/2
  Product/1 -> Add1/1, Add/1
  ProducT1/1 -> Add1/2, Add/2
  Add/1 -> Uref2/1
  Add1/1 -> Uref3/1

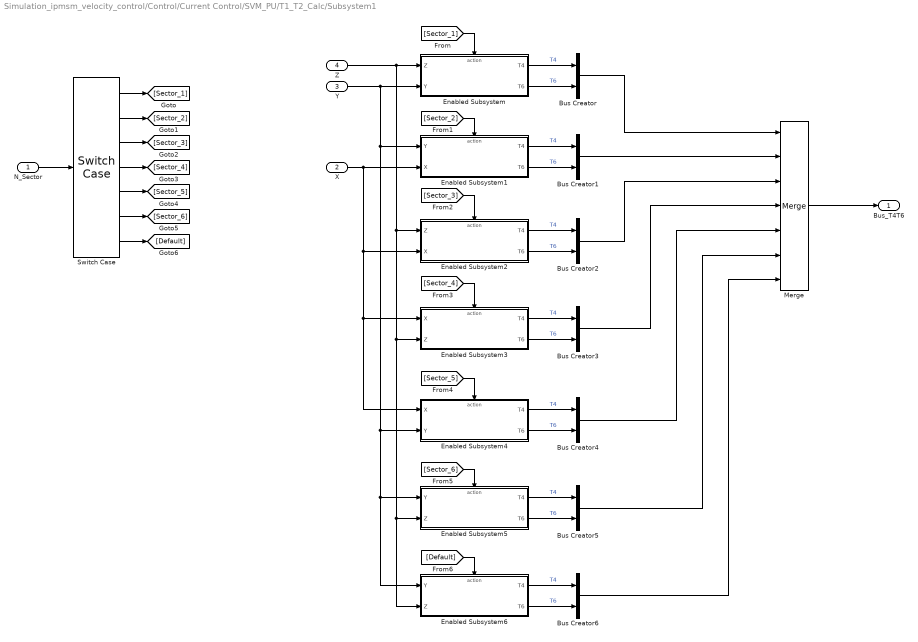
== system Simulation_ipmsm_velocity_control/Control/Current Control/SVM_PU/T1_T2_Calc/Subsystem1 ==
  N_Sector : Inport
  X : Inport  Port=2
  Y : Inport  Port=3
  Z : Inport  Port=4
  Bus Creator{,1..6} (7 alike) : BusCreator  Inputs=2
  Enabled Subsystem : Subsystem  TreatAsAtomicUnit=on
  Enabled Subsystem1 : Subsystem  TreatAsAtomicUnit=on
  Enabled Subsystem2 : Subsystem  TreatAsAtomicUnit=on
  Enabled Subsystem3 : Subsystem  TreatAsAtomicUnit=on
  Enabled Subsystem4 : Subsystem  TreatAsAtomicUnit=on
  Enabled Subsystem5 : Subsystem  TreatAsAtomicUnit=on
  Enabled Subsystem6 : Subsystem  TreatAsAtomicUnit=on
  Merge : Merge  Inputs=7
  Switch Case : SwitchCase  CaseConditions={1,2,3,4,5,6}
  Bus_T4T6 : Outport
  wires:
  N_Sector/1 -> Switch Case/1
  Switch Case/1 -> [Sector_1]
  Switch Case/2 -> [Sector_2]
  Switch Case/3 -> [Sector_3]
  Switch Case/4 -> [Sector_4]
  Switch Case/5 -> [Sector_5]
  Switch Case/6 -> [Sector_6]
  Switch Case/7 -> [Default]
  [Sector_1] -> Enabled Subsystem/Action
  Y/1 -> Enabled Subsystem6/1(Y), Enabled Subsystem5/1(Y), Enabled Subsystem4/2(Y), Enabled Subsystem1/1(Y), Enabled Subsystem/2(Y)
  Z/1 -> Enabled Subsystem3/2(Z), Enabled Subsystem6/2(Z), Enabled Subsystem5/2(Z), Enabled Subsystem2/1(Z), Enabled Subsystem/1(Z)
  [Sector_2] -> Enabled Subsystem1/Action
  X/1 -> Enabled Subsystem4/1(X), Enabled Subsystem3/1(X), Enabled Subsystem2/2(X), Enabled Subsystem1/2(X)
  [Sector_3] -> Enabled Subsystem2/Action
  [Sector_4] -> Enabled Subsystem3/Action
  [Sector_5] -> Enabled Subsystem4/Action
  [Sector_6] -> Enabled Subsystem5/Action
  [Default] -> Enabled Subsystem6/Action
  Enabled Subsystem/1(T4) -> Bus Creator/1  "T4"
  Enabled Subsystem/2(T6) -> Bus Creator/2  "T6"
  Enabled Subsystem1/2(T6) -> Bus Creator1/2  "T6"
  Enabled Subsystem1/1(T4) -> Bus Creator1/1  "T4"
  Enabled Subsystem2/1(T4) -> Bus Creator2/1  "T4"
  Enabled Subsystem3/1(T4) -> Bus Creator3/1  "T4"
  Enabled Subsystem2/2(T6) -> Bus Creator2/2  "T6"
  Enabled Subsystem3/2(T6) -> Bus Creator3/2  "T6"
  Enabled Subsystem4/1(T4) -> Bus Creator4/1  "T4"
  Enabled Subsystem5/1(T4) -> Bus Creator5/1  "T4"
  Enabled Subsystem4/2(T6) -> Bus Creator4/2  "T6"
  Enabled Subsystem5/2(T6) -> Bus Creator5/2  "T6"
  Enabled Subsystem6/1(T4) -> Bus Creator6/1  "T4"
  Enabled Subsystem6/2(T6) -> Bus Creator6/2  "T6"
  Bus Creator/1 -> Merge/1
  Bus Creator1/1 -> Merge/2
  Bus Creator2/1 -> Merge/3
  Bus Creator3/1 -> Merge/4
  Bus Creator4/1 -> Merge/5
  Bus Creator5/1 -> Merge/6
  Bus Creator6/1 -> Merge/7
  Merge/1 -> Bus_T4T6/1

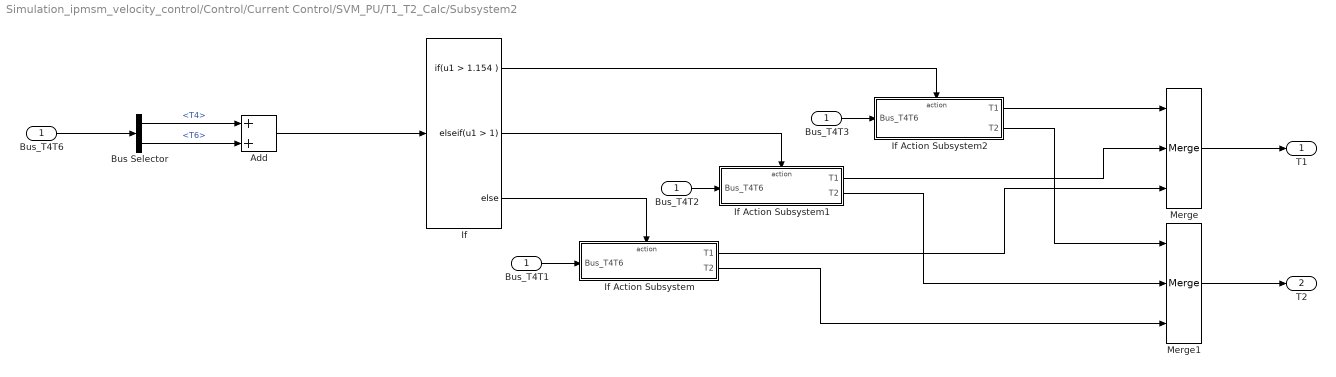
== system Simulation_ipmsm_velocity_control/Control/Current Control/SVM_PU/T1_T2_Calc/Subsystem2 ==
  Bus_T4T6 : Inport
  Add : Sum
  Bus Selector : BusSelector  OutputSignals=T4,T6
  Bus_T4T1 : InportShadow
  Bus_T4T2 : InportShadow
  Bus_T4T3 : InportShadow
  If : If  IfExpression=u1 > 1.154  ElseIfExpressions=u1 > 1
  If Action Subsystem : Subsystem  TreatAsAtomicUnit=on
  If Action Subsystem1 : Subsystem  TreatAsAtomicUnit=on
  If Action Subsystem2 : Subsystem  TreatAsAtomicUnit=on
  Merge : Merge  Inputs=3
  Merge1 : Merge  Inputs=3
  T1 : Outport
  T2 : Outport  Port=2
  wires:
  Bus_T4T6/1 -> Bus Selector/1
  Bus Selector/1 -> Add/1  "<T4>"
  Bus Selector/2 -> Add/2  "<T6>"
  Add/1 -> If/1
  If/3 -> If Action Subsystem/Action
  If/2 -> If Action Subsystem1/Action
  If/1 -> If Action Subsystem2/Action
  Bus_T4T1/1 -> If Action Subsystem/1(Bus_T4T6)
  Bus_T4T2/1 -> If Action Subsystem1/1(Bus_T4T6)
  Bus_T4T3/1 -> If Action Subsystem2/1(Bus_T4T6)
  Merge/1 -> T1/1
  If Action Subsystem2/1(T1) -> Merge/1
  If Action Subsystem1/1(T1) -> Merge/2
  If Action Subsystem/1(T1) -> Merge/3
  If Action Subsystem2/2(T2) -> Merge1/1
  If Action Subsystem1/2(T2) -> Merge1/2
  If Action Subsystem/2(T2) -> Merge1/3
  Merge1/1 -> T2/1

== system Simulation_ipmsm_velocity_control/Control/Current Control/SVM_PU/T1_T2_Calc/T4_T6 ==
  T4 : Inport
  T6 : Inport  Port=2
  Add : Sum
  Divide : Product  Inputs=*/
  Divide1 : Product  Inputs=*/
  Mux : Mux  Inputs=2
  Mux1 : Mux  Inputs=2
  Switch : Switch  Criteria=u2 > Threshold  Threshold=1  SaturateOnIntegerOverflow=off  InputSameDT=off
  T4_T6 : Outport
  wires:
  T4/1 -> Add/1, Mux1/1, Divide/1
  T6/1 -> Mux1/2, Add/2, Divide1/1
  Add/1 -> Divide1/2, Divide/2, Switch/2
  Divide/1 -> Mux/1  "T4"
  Divide1/1 -> Mux/2  "T6"
  Mux/1 -> Switch/1
  Mux1/1 -> Switch/3
  Switch/1 -> T4_T6/1

== system Simulation_ipmsm_velocity_control/Control/Current Control/SVM_PU/Tcm_Calc/If Action Subsystem ==
  Ta : Inport
  Tb : Inport  Port=2
  Tc : Inport  Port=3
  Action Port : ActionPort  ActionPortLabel=case [ 1 ]:
  Tcm1 : Outport
  Tcm2 : Outport  Port=2
  Tcm3 : Outport  Port=3
  wires:
  Tb/1 -> Tcm1/1
  Ta/1 -> Tcm2/1
  Tc/1 -> Tcm3/1

== system Simulation_ipmsm_velocity_control/Control/Current Control/SVM_PU/Tcm_Calc/If Action Subsystem1 ==
  Ta : Inport
  Tb : Inport  Port=2
  Tc : Inport  Port=3
  Action Port : ActionPort  ActionPortLabel=case [ 3 ]:
  Tcm1 : Outport
  Tcm2 : Outport  Port=2
  Tcm3 : Outport  Port=3
  wires:
  Ta/1 -> Tcm1/1
  Tb/1 -> Tcm2/1
  Tc/1 -> Tcm3/1

== system Simulation_ipmsm_velocity_control/Control/Current Control/SVM_PU/Tcm_Calc/If Action Subsystem2 ==
  Ta : Inport
  Tb : Inport  Port=2
  Tc : Inport  Port=3
  Action Port : ActionPort  ActionPortLabel=case [ 4 ]:
  Tcm1 : Outport
  Tcm2 : Outport  Port=2
  Tcm3 : Outport  Port=3
  wires:
  Tc/1 -> Tcm1/1
  Tb/1 -> Tcm2/1
  Ta/1 -> Tcm3/1

== system Simulation_ipmsm_velocity_control/Control/Current Control/SVM_PU/Tcm_Calc/If Action Subsystem3 ==
  Ta : Inport
  Tb : Inport  Port=2
  Tc : Inport  Port=3
  Action Port : ActionPort  ActionPortLabel=case [ 5 ]:
  Tcm1 : Outport
  Tcm2 : Outport  Port=2
  Tcm3 : Outport  Port=3
  wires:
  Tc/1 -> Tcm1/1
  Tb/1 -> Tcm3/1
  Ta/1 -> Tcm2/1

== system Simulation_ipmsm_velocity_control/Control/Current Control/SVM_PU/Tcm_Calc/If Action Subsystem4 ==
  Ta : Inport
  Tb : Inport  Port=2
  Tc : Inport  Port=3
  Action Port : ActionPort  ActionPortLabel=case [ 6 ]:
  Tcm1 : Outport
  Tcm2 : Outport  Port=2
  Tcm3 : Outport  Port=3
  wires:
  Tc/1 -> Tcm2/1
  Tb/1 -> Tcm1/1
  Ta/1 -> Tcm3/1

== system Simulation_ipmsm_velocity_control/Control/Current Control/SVM_PU/Tcm_Calc/If Action Subsystem5 ==
  Ta : Inport
  Tb : Inport  Port=2
  Tc : Inport  Port=3
  Action Port : ActionPort  ActionPortLabel=default:
  Tcm1 : Outport
  Tcm2 : Outport  Port=2
  Tcm3 : Outport  Port=3
  wires:
  Tc/1 -> Tcm2/1
  Tb/1 -> Tcm1/1
  Ta/1 -> Tcm3/1

== system Simulation_ipmsm_velocity_control/Control/Current Control/SVM_PU/Tcm_Calc/If Action Subsystem7 ==
  Ta : Inport
  Tb : Inport  Port=2
  Tc : Inport  Port=3
  Action Port : ActionPort  ActionPortLabel=case [ 2 ]:
  Tcm1 : Outport
  Tcm2 : Outport  Port=2
  Tcm3 : Outport  Port=3
  wires:
  Ta/1 -> Tcm1/1
  Tc/1 -> Tcm2/1
  Tb/1 -> Tcm3/1
